simulink model "DataLoggerRefMod"  (R2016b)
settings: Solver=VariableStepAuto  StartTime=0.0  StopTime=10.0  RelTol=1e-3
settings Model: DataDictionary=DataDictionary.sldd  Creator=Taeke  LastModifiedBy=Taeke
settings ModelReferenceCC: ModelReferenceNumInstancesAllowed=Single

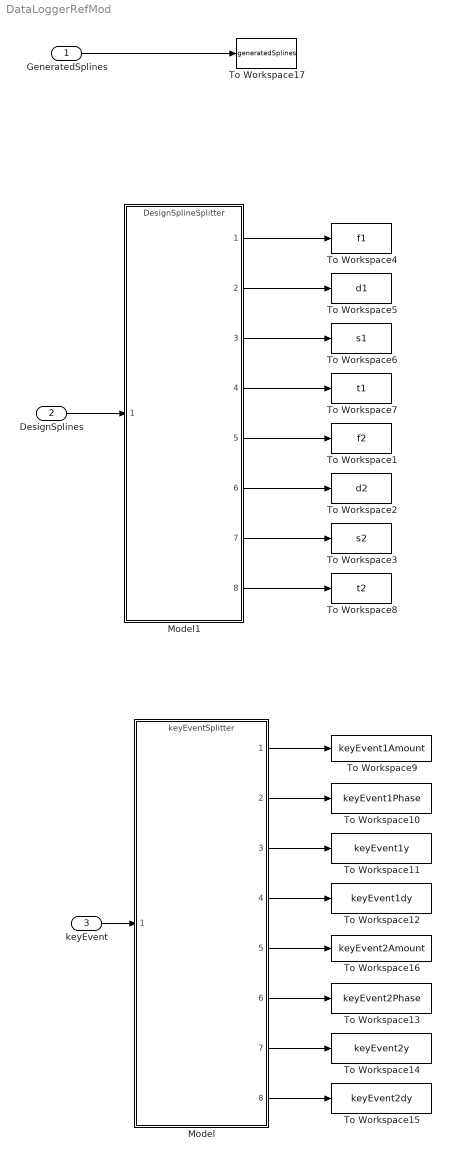
== system DataLoggerRefMod ==
  GeneratedSplines : Inport  OutDataTypeStr=Bus: generatedSplines
  DesignSplines : Inport  Port=2  OutDataTypeStr=Bus: designSplineTotal
  keyEvent : Inport  Port=3  OutDataTypeStr=Bus: keyEventTotal
  Model : ModelReference  ModelNameDialog=keyEventSplitter.slx  SimulationMode=Normal  ModelReferenceVersion=1.3
  Model1 : ModelReference  ModelNameDialog=DesignSplineSplitter.slx  SimulationMode=Normal  ModelReferenceVersion=1.4
  To Workspace1 : ToWorkspace  VariableName=f2  SaveFormat=Timeseries  SampleTime=-1
  To Workspace10 : ToWorkspace  VariableName=keyEvent1Phase  SaveFormat=Timeseries  SampleTime=-1
  To Workspace11 : ToWorkspace  VariableName=keyEvent1y  SaveFormat=Timeseries  SampleTime=-1
  To Workspace12 : ToWorkspace  VariableName=keyEvent1dy  SaveFormat=Timeseries  SampleTime=-1
  To Workspace13 : ToWorkspace  VariableName=keyEvent2Phase  SaveFormat=Timeseries  SampleTime=-1
  To Workspace14 : ToWorkspace  VariableName=keyEvent2y  SaveFormat=Timeseries  SampleTime=-1
  To Workspace15 : ToWorkspace  VariableName=keyEvent2dy  SaveFormat=Timeseries  SampleTime=-1
  To Workspace16 : ToWorkspace  VariableName=keyEvent2Amount  SaveFormat=Timeseries  SampleTime=-1
  To Workspace17 : ToWorkspace  VariableName=generatedSplines  SaveFormat=Timeseries  SampleTime=-1
  To Workspace2 : ToWorkspace  VariableName=d2  SaveFormat=Timeseries  SampleTime=-1
  To Workspace3 : ToWorkspace  VariableName=s2  SaveFormat=Timeseries  SampleTime=-1
  To Workspace4 : ToWorkspace  VariableName=f1  SaveFormat=Timeseries  SampleTime=-1
  To Workspace5 : ToWorkspace  VariableName=d1  SaveFormat=Timeseries  SampleTime=-1
  To Workspace6 : ToWorkspace  VariableName=s1  SaveFormat=Timeseries  SampleTime=-1
  To Workspace7 : ToWorkspace  VariableName=t1  SaveFormat=Timeseries  SampleTime=-1
  To Workspace8 : ToWorkspace  VariableName=t2  SaveFormat=Timeseries  SampleTime=-1
  To Workspace9 : ToWorkspace  VariableName=keyEvent1Amount  SaveFormat=Timeseries  SampleTime=-1
  wires:
  Model1/1 -> To Workspace4/1
  Model1/2 -> To Workspace5/1
  Model1/3 -> To Workspace6/1
  Model1/4 -> To Workspace7/1
  Model1/5 -> To Workspace1/1
  Model1/6 -> To Workspace2/1
  Model1/7 -> To Workspace3/1
  Model1/8 -> To Workspace8/1
  keyEvent/1 -> Model/1
  Model/1 -> To Workspace9/1
  Model/2 -> To Workspace10/1
  Model/3 -> To Workspace11/1
  Model/4 -> To Workspace12/1
  Model/5 -> To Workspace16/1
  Model/6 -> To Workspace13/1
  Model/7 -> To Workspace14/1
  Model/8 -> To Workspace15/1
  DesignSplines/1 -> Model1/1
  GeneratedSplines/1 -> To Workspace17/1
